simulink model "Teleop_simulation"  (R2021a)
settings: Solver=VariableStepAuto  StartTime=0.0  StopTime=inf  RelTol=1e-3
undefined symbols (not defined in the file): Force, Position
libraries: robotlib x8, vrlib x1, dspinverses x1, dspmathops x1
settings Model: Creator=workcell  LastModifiedBy=workcell

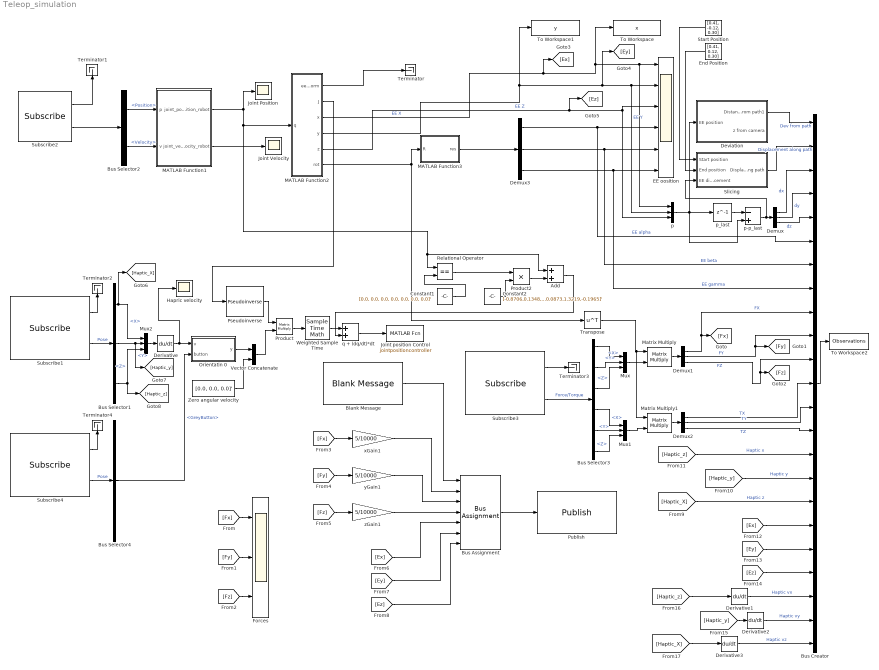
== system Teleop_simulation ==
  Add : Sum
  Blank Message : robotlib/Blank Message  messageClass=Message  entityType=omni_msgs/OmniFeedback  messageType=omni_msgs/OmniFeedback  SampleTime=inf  legacyBusStruct=off
  Bus Assignment : BusAssignment  AssignedSignals=Force.X,Force.Y,Force.Z,Position.Z,Position.Y,Position.X
  Bus Creator : BusCreator  Inputs=23
  Bus Selector1 : BusSelector  OutputSignals=Pose.Position.X,Pose.Position.Y,Pose.Position.Z
  Bus Selector2 : BusSelector  OutputSignals=Position,Velocity
  Bus Selector3 : BusSelector  OutputSignals=Wrench.Force.X,Wrench.Force.Y,Wrench.Force.Z,Wrench.Torque.X,Wrench.Torque.Y,Wrench.Torque.Z
  Bus Selector4 : BusSelector  OutputSignals=GreyButton
  Constant1 : Constant  Value=[0.0, 0.0, 0.0, 0.0, 0.0, 0.0, 0.0]'
  Constant2 : Constant  Value=[-0.8706,0.1348,0.6560,-1.7221,-0.0873,1.3219,-0.1965]'
  Demux{,1..3} (4 alike) : Demux  Outputs=3
  Derivative{,1..3} (4 alike) : Derivative
  Deviation : Subsystem
  EE oosition : Scope  NumInputPorts=6
  End Position : Constant  Value=[0.41, 0.12, 0.30]  VectorParams1D=off
  Forces : Scope  NumInputPorts=3
  Hapric velocity : Scope
  Joint Position : Scope
  Joint Velocity : Scope
  Joint position Control : MATLABFcn  MATLABFcn=jointpositioncontroller  OutputDimensions=0
  MATLAB Function1 : MATLAB Function  TreatAsAtomicUnit=on
  MATLAB Function2 : MATLAB Function  TreatAsAtomicUnit=on
  MATLAB Function3 : MATLAB Function  TreatAsAtomicUnit=on
  Matrix Multiply : Product  Multiplication=Matrix(*)
  Matrix Multiply1 : Product  Multiplication=Matrix(*)
  Mux : Mux  Inputs=3
  Mux1 : Mux  Inputs=3
  Mux2 : Mux  Inputs=3
  Orientatin 0 : MATLAB Function  TreatAsAtomicUnit=on
  Product : Product  Multiplication=Matrix(*)
  Product2 : Product
  Pseudoinverse : dspinverses/Pseudoinverse  wanterr=off  SimulateUsing=Interpreted execution
      settings: SourceProductBaseCode=DS
  Publish : robotlib/Publish  topicSource=Select from ROS network  topic=/phantom/force_feedback  messageType=omni_msgs/OmniFeedback  legacyBusStruct=off  messageQueueLength=1
  Relational Operator : RelationalOperator  Operator===  OutDataTypeStr=boolean  RndMeth=Simplest
  Slicing : Subsystem
  Start Position : Constant  Value=[0.41, -0.12, 0.30]  VectorParams1D=off
  Subscribe1 : robotlib/Subscribe  topicSource=Select from ROS network  topic=/phantom/pose  messageType=geometry_msgs/PoseStamped  SampleTime=-1  legacyBusStruct=off  messageQueueLength=1
  Subscribe2 : robotlib/Subscribe  topicSource=Select from ROS network  topic=/iiwa/joint_states  messageType=sensor_msgs/JointState  SampleTime=-1  legacyBusStruct=off  messageQueueLength=1
  Subscribe3 : robotlib/Subscribe  topicSource=Select from ROS network  topic=/iiwa/CartesianWrench  messageType=geometry_msgs/WrenchStamped  SampleTime=-1  legacyBusStruct=off  messageQueueLength=1
  Subscribe4 : robotlib/Subscribe  topicSource=Select from ROS network  topic=/phantom/button  messageType=omni_msgs/OmniButtonEvent  SampleTime=-1  legacyBusStruct=off  messageQueueLength=1
  Terminator{,1..4} (5 alike) : Terminator
  To Workspace : ToWorkspace  VariableName=x  SaveFormat=Timeseries  SampleTime=-1
  To Workspace1 : ToWorkspace  VariableName=y  SaveFormat=Timeseries  SampleTime=-1
  To Workspace2 : ToWorkspace  VariableName=Observations  SaveFormat=Timeseries  SampleTime=-1
  Transpose : Math  Operator=transpose  SaturateOnIntegerOverflow=on
  Vector Concatenate : Concatenate
  Weighted Sample Time : SampleTimeMath  TsampMathOp=*
  Zero angular velocity : Constant  Value=[0.0, 0.0, 0.0]'
  p : Mux  Inputs=3
  p-p_last : Sum  Inputs=-+
  p_last : Delay  DelayLength=1  InitialCondition=0
  q + (dq/dt)*dt : Sum
  xGain1 : Gain  Gain=5/10000
  yGain1 : Gain  Gain=5/10000
  zGain1 : Gain  Gain=5/10000
  wires:
  Transpose/1 -> Matrix Multiply1/1, Matrix Multiply/1
  Demux2/2 -> Bus Creator/13  "TY"
  Matrix Multiply1/1 -> Demux2/1
  Demux2/3 -> Bus Creator/14  "TZ"
  Subscribe2/2 -> Bus Selector2/1
  Bus Selector3/2 -> Mux/2  "<Y>"
  Bus Selector3/6 -> Mux1/3  "<Z>"
  Demux/3 -> Bus Creator/5  "dz"
  q + (dq/dt)*dt/1 -> Joint position Control/1
  Bus Selector3/4 -> Mux1/1  "<X>"
  Deviation/1(Distance from path1) -> Bus Creator/1  "Dev from path"
  MATLAB Function1/2(joint_velocity_robot) -> Joint Velocity/1
  MATLAB Function2/6(rot) -> MATLAB Function3/1(R), Transpose/1
  Mux1/1 -> Matrix Multiply1/2
  MATLAB Function2/4(y) -> [Ey], EE oosition/2, p/2, To Workspace1/1  "EE Y"
  Subscribe2/1 -> Terminator1/1
  Relational Operator/1 -> Product2/1
  Bus Selector2/1 -> MATLAB Function1/1(p)  "<Position>"
  Product2/1 -> Add/2
  Start Position/1 -> Slicing/1(Start position)
  Bus Selector2/2 -> MATLAB Function1/2(v)  "<Velocity>"
  Demux3/1 -> Bus Creator/6, EE oosition/4  "EE alpha"
  Bus Selector3/5 -> Mux1/2  "<Y>"
  Demux/2 -> Bus Creator/4  "dy"
  Constant2/1 -> Product2/2
  p_last/1 -> p-p_last/1
  Subscribe3/2 -> Bus Selector3/1  "Force/Torque"
  Demux2/1 -> Bus Creator/12  "TX"
  Demux1/3 -> [Fz], Bus Creator/11  "FZ"
  MATLAB Function2/3(x) -> [Ex], To Workspace/1, EE oosition/1, p/1  "EE X"
  MATLAB Function2/2(J) -> Pseudoinverse/1
  Demux3/3 -> Bus Creator/8, EE oosition/6  "EE gamma"
  MATLAB Function2/1(eef_transform) -> Terminator/1
  Pseudoinverse/1 -> Product/1
  MATLAB Function2/5(z) -> [Ez], EE oosition/3, p/3  "EE Z"
  MATLAB Function3/1(res) -> Demux3/1
  Zero angular velocity/1 -> Vector Concatenate/2
  Demux/1 -> Bus Creator/3  "dx"
  Demux3/2 -> Bus Creator/7, EE oosition/5  "EE beta"
  Slicing/1(Displacement along path) -> Bus Creator/2  "Displacement along path"
  p-p_last/1 -> Slicing/3(EE displacement), Demux/1
  p/1 -> Deviation/1(EE position), p-p_last/2, p_last/1
  Subscribe3/1 -> Terminator3/1
  Constant1/1 -> Relational Operator/2
  MATLAB Function1/1(joint_position_robot) -> Relational Operator/1, Add/1, MATLAB Function2/1(q), Joint Position/1
  Bus Selector3/1 -> Mux/1  "<X>"
  Demux1/1 -> [Fx], Bus Creator/9  "FX"
  Demux1/2 -> [Fy], Bus Creator/10  "FY"
  Bus Selector3/3 -> Mux/3  "<Z>"
  Mux/1 -> Matrix Multiply/2
  Add/1 -> q + (dq/dt)*dt/2
  Weighted Sample Time/1 -> q + (dq/dt)*dt/1
  End Position/1 -> Slicing/2(End position)
  Product/1 -> Weighted Sample Time/1
  Matrix Multiply/1 -> Demux1/1
  Subscribe1/2 -> Bus Selector1/1  "Pose"
  Bus Selector1/1 -> Mux2/1, [Haptic_X]  "<X>"
  Bus Selector1/2 -> [Haptic_y], Mux2/2  "<Y>"
  Bus Selector1/3 -> [Haptic_z], Mux2/3  "<Z>"
  Mux2/1 -> Derivative/1
  Subscribe1/1 -> Terminator2/1
  Bus Creator/1 -> To Workspace2/1
  Subscribe4/2 -> Bus Selector4/1  "Pose"
  Subscribe4/1 -> Terminator4/1
  Bus Selector4/1 -> Orientatin 0/2(button)  "<GreyButton>"
  Derivative/1 -> Hapric velocity/1, Orientatin 0/1(v)
  Orientatin 0/1(y) -> Vector Concatenate/1
  Blank Message/1 -> Bus Assignment/1
  Bus Assignment/1 -> Publish/1
  xGain1/1 -> Bus Assignment/2
  yGain1/1 -> Bus Assignment/3
  zGain1/1 -> Bus Assignment/4
  [Fz] -> zGain1/1
  [Fx] -> xGain1/1
  [Fy] -> yGain1/1
  [Ex] -> Bus Assignment/5
  [Ey] -> Bus Assignment/6
  [Ez] -> Bus Assignment/7
  Vector Concatenate/1 -> Product/2
  [Fx] -> Forces/1
  [Fy] -> Forces/2
  [Fz] -> Forces/3
  [Haptic_z] -> Bus Creator/15  "Haptic x"
  [Haptic_y] -> Bus Creator/16  "Haptic y"
  [Haptic_X] -> Bus Creator/17  "Haptic z"
  [Ex] -> Bus Creator/18
  [Ey] -> Bus Creator/19
  [Ez] -> Bus Creator/20
  [Haptic_z] -> Derivative1/1
  [Haptic_X] -> Derivative3/1
  [Haptic_y] -> Derivative2/1
  Derivative1/1 -> Bus Creator/21  "Haptic vx"
  Derivative2/1 -> Bus Creator/22  "Haptic vy"
  Derivative3/1 -> Bus Creator/23  "Haptic vz"

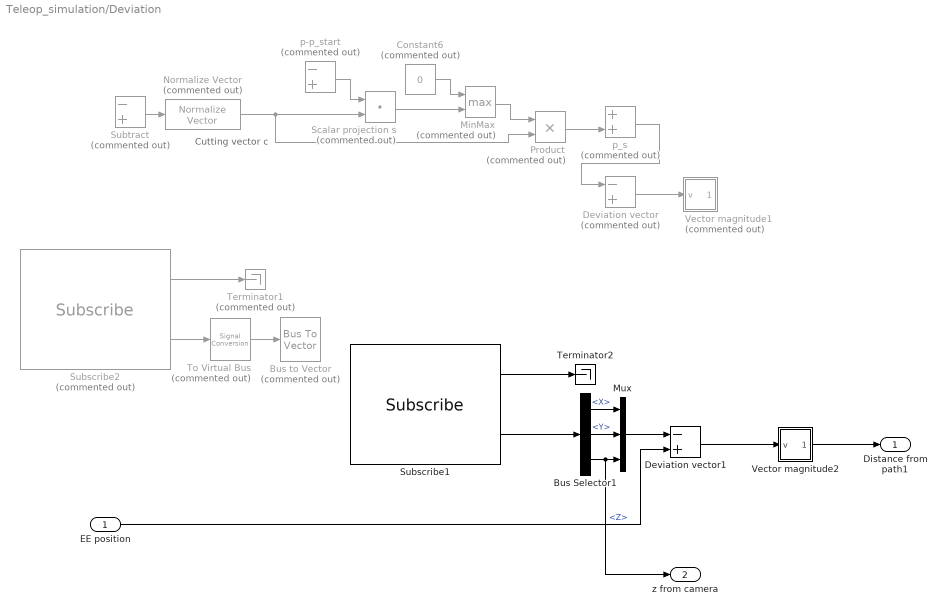
== system Teleop_simulation/Deviation ==
  note: Cutting vector c
  EE position : Inport
  Bus Selector1 : BusSelector  OutputSignals=Pose.Position.X,Pose.Position.Y,Pose.Position.Z
  Bus to Vector : BusToVector  Commented=on
  Constant6 : Constant  Commented=on  Value=0
  Deviation vector : Sum  Commented=on  Inputs=-+
  Deviation vector1 : Sum  Inputs=-+
  MinMax : MinMax  Commented=on  Function=max  Inputs=2  OutMin=[0]
  Mux : Mux  Inputs=3
  Normalize Vector : vrlib/Utilities/Normalize Vector  Commented=on  maxzero=0
  Product : Product  Commented=on
  Scalar projection s : DotProduct  Commented=on  InputSameDT=on  OutDataTypeStr=Inherit: Inherit via internal rule
  Subscribe1 : robotlib/Subscribe  topicSource=Select from ROS network  topic=/iiwa/CartesianPose/surface  messageType=geometry_msgs/PoseStamped  SampleTime=-1  legacyBusStruct=off  messageQueueLength=1
  Subscribe2 : robotlib/Subscribe  Commented=on  topicSource=Select from ROS network  topic=/iiwa/CartesianPose/surface  messageType=geometry_msgs/PoseStamped  SampleTime=-1  legacyBusStruct=off  messageQueueLength=1
  Subtract : Sum  Commented=on  Inputs=-+
  Terminator1 : Terminator  Commented=on
  Terminator2 : Terminator
  To Virtual Bus : SignalConversion  Commented=on  ConversionOutput=Virtual bus  OverrideOpt=off
  Vector magnitude1 : Subsystem  Commented=on
  Vector magnitude2 : Subsystem
  p-p_start : Sum  Commented=on  Inputs=-+
  p_s : Sum  Commented=on
  Distance from path1 : Outport
  z from camera : Outport  Port=2
  wires:
  Product/1 -> p_s/2
  Subtract/1 -> Normalize Vector/1
  p-p_start/1 -> Scalar projection s/1
  Scalar projection s/1 -> MinMax/2
  Constant6/1 -> MinMax/1
  MinMax/1 -> Product/1
  p_s/1 -> Deviation vector/1
  Normalize Vector/1 -> Product/2, Scalar projection s/2
  Deviation vector/1 -> Vector magnitude1/1(v)
  EE position/1 -> Deviation vector1/2
  Vector magnitude2/1(||v||) -> Distance from path1/1
  Subscribe2/1 -> Terminator1/1
  To Virtual Bus/1 -> Bus to Vector/1
  Subscribe2/2 -> To Virtual Bus/1
  Mux/1 -> Deviation vector1/1
  Subscribe1/1 -> Terminator2/1
  Bus Selector1/1 -> Mux/1  "<X>"
  Subscribe1/2 -> Bus Selector1/1
  Bus Selector1/2 -> Mux/2  "<Y>"
  Deviation vector1/1 -> Vector magnitude2/1(v)
  Bus Selector1/3 -> z from camera/1, Mux/3  "<Z>"

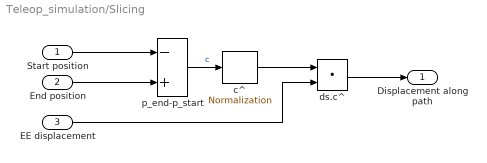
== system Teleop_simulation/Slicing ==
  Start position : Inport
  End position : Inport  Port=2
  EE displacement : Inport  Port=3
  c^ : dspmathops/Normalization  NormType=2-norm  Bias=1e-10  NormOver=Each column  Dimension=1  roundingMode=Floor  overflowMode=off  accumDataTypeStr=Inherit: Same as product output  accumLastDataTypeStr=Inherit: Same as product output  outputDataTypeStr=Inherit: Same as product output  outputMin=[]  outputMax=[]  outputLastDataTypeStr=Inherit: Same as product output
  ds.c^ : DotProduct  InputSameDT=on  OutDataTypeStr=Inherit: Inherit via internal rule
  p_end-p_start : Sum  Inputs=-+
  Displacement along path : Outport
  wires:
  Start position/1 -> p_end-p_start/1
  End position/1 -> p_end-p_start/2
  p_end-p_start/1 -> c^/1  "c"
  EE displacement/1 -> ds.c^/2
  c^/1 -> ds.c^/1
  ds.c^/1 -> Displacement along path/1

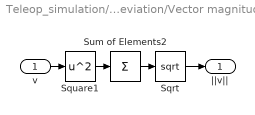
== system Teleop_simulation/Deviation/Vector magnitude1 ==
  v : Inport
  Sqrt : Sqrt  SaturateOnIntegerOverflow=on
  Square1 : Math  Operator=square  SaturateOnIntegerOverflow=on
  Sum of Elements2 : Sum  Inputs=+
  ||v|| : Outport
  wires:
  Sqrt/1 -> ||v||/1
  Sum of Elements2/1 -> Sqrt/1
  Square1/1 -> Sum of Elements2/1
  v/1 -> Square1/1

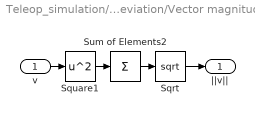
== system Teleop_simulation/Deviation/Vector magnitude2 ==
  v : Inport
  Sqrt : Sqrt  SaturateOnIntegerOverflow=on
  Square1 : Math  Operator=square  SaturateOnIntegerOverflow=on
  Sum of Elements2 : Sum  Inputs=+
  ||v|| : Outport
  wires:
  Sqrt/1 -> ||v||/1
  Sum of Elements2/1 -> Sqrt/1
  Square1/1 -> Sum of Elements2/1
  v/1 -> Square1/1

== matlab function Teleop_simulation/MATLAB Function2 ==
  data: q input; eef_transform output; J output; x output; y output; z output; rot output
%function [eef_transform,J,x,y,z,rot]=directKinematics(q1,q2,q3,q4,q5,q6,q7)
function [eef_transform,J,x,y,z,rot]=directKinematics(q)
% DH PARAMETERS FOR THE ROBOT
alfa={0,-pi/2,pi/2,pi/2,-pi/2,-pi/2,pi/2};
%q=[q1,q2,q3,q4,q5,q6,q7];
d={0.36,0.0,0.42,0.0,0.4,0.0,0.126};
d{7}=0.020+0.34017; 
a={0,0,0,0,0,0,0};

%% Calculating the direct Kinematics
T=zeros(4,4,7);
i=1;
T(:,:,i)=getDHMatrix(alfa{i},q(i),d{i},a{i});
    for i=2:7
        T(:,:,i)=T(:,:,i-1)*getDHMatrix(alfa{i},q(i),d{i},a{i});
        T(:,:,i)=normalizeColumns(T(:,:,i));
    end
        T(:,:,7)=T(:,:,7);
        T(:,:,7)=normalizeColumns(T(:,:,7));
        
    pef=T(1:3,4,7);
    J=zeros(6,7);
    for i=1:7
        k=T(1:3,3,i);
        pij=pef-T(1:3,4,i);
        J(1:3,i)=cross(k,pij);
        J(4:6,i)=k;
    end
%% End effector transform
eef_transform=T(:,:,7);
x=T(1,4,7);
y=T(2,4,7);
z=T(3,4,7);
rot=T(1:3,1:3,7);
end

function T=getDHMatrix(alfa,theta,d,a)
T=zeros(4,4);
calpha=cos(alfa);
sinalpha=sin(alfa);
coshteta=cos(theta);
sintheta=sin(theta);

T(1,1)=coshteta;
T(2,1)=sintheta*calpha;
T(3,1)=sintheta*sinalpha;				

T(1,2)=-sintheta;
T(2,2)=coshteta*calpha;
T(3,2)=coshteta*sinalpha;

T(2,3)=-sinalpha;
T(3,3)=calpha;

T(1,4)=a;
T(2,4)=-sinalpha*d;
T(3,4)=calpha*d;
T(4,4)=1;

end

function normalizedT=normalizeColumns(T)

r=zeros(4,3); % corrected rotatio matrix, with zero badding row at the end
for j=1:3
    r(1:3,j)=T(1:3,j)/norm(T(1:3,j));
end
normalizedT=[r,T(:,4)];
end

== matlab function Teleop_simulation/Orientatin 0 ==
  data: v input; y output; button input
function y = fcn(v, button)

if button == 1    
    %y = smoothdata(v,'gaussian'); 
   % y = lowpass(v,500);
    y = v;
else
y = [0,0,0]';
end

== matlab function Teleop_simulation/MATLAB Function3 ==
  data: R input; res output
function res=rot2eulZYX(R)
    [res]=eulerAngles(R) ;
end

function y=closeEnough(a,b)
    epsilon=0.000001;
    if (epsilon>abs(a-b))
        y=1;
    else
        y=0;
    end
end

function [res]=eulerAngles(R) 
    %% check for gimbal lock
    R=R';
    if (closeEnough(R(1,3), -1.0)) 
        b = 0; %% gimbal lock, value of x doesn't matter
        c = pi / 2;
        a = b + atan2(R(2,1), R(3,1));
    elseif (closeEnough(R(1,3), 1.0)) 
        b = 0;
        c = -pi / 2;
        a = -b + atan2(-R(2,1), -R(3,1));
    else  %% two solutions exist
        b1 = -asin(R(1,3));
        b2 = pi - b1;

        c1 = atan2(R(2,3) / cos(b1), R(3,3) / cos(b1));
        c2 = atan2(R(2,3) / cos(b2), R(3,3) / cos(b2));

        a1 = atan2(R(1,2) / cos(b1), R(1,1)/ cos(b1));
        a2 = atan2(R(1,2) / cos(b2), R(1,1) / cos(b2));

        %% choose one solution to return
        %% for example the "shortest" rotation
        condition=((abs(b1) + abs(c1) + abs(a1)) <= (abs(b2) + abs(c2) + abs(a2)));
        if condition 
            a=a1;
            b=b1;
            c=c1;   
        else 
            a=a2;
            b=b2;
            c=c2;   
        end
    end
    res=[a,b,c];
end

== matlab function Teleop_simulation/MATLAB Function1 ==
  data: joint_position_robot output; joint_velocity_robot output; p input; v input
function  [joint_position_robot,joint_velocity_robot]=states(p,v)
joint_position_robot=[p(1),p(2),p(3),p(4),p(5),p(6),p(7)]';
joint_velocity_robot=[v(1),v(2),v(3),v(4),v(5),v(6),v(7)]';         
end
